simulink model "raibert_controller_1_3"  (R2018b)
settings: Solver=FixedStepDiscrete  StartTime=0.0  StopTime=inf  FixedStep=sample_time  RelTol=1e-3
InitFcn:
  | raibert_controller_params_1_3
  | warning off all
values from neighbouring files (symbols this model uses):
  sample_time = 1/sample_freq    (= 0.001)    [simulation_params.m]
undefined symbols (not defined in the file or in its folder): ctrl, Discrete, initial_dx_estimate, initial_dy_estimate, initial_dz_estimate, initial_z_estimate, Time
libraries: simulink x30, ctrlSharedLib x7
(part 1 of 4)
settings Model: Creator=wmartin  LastModifiedBy=akhadke
settings DataIOCC: SaveFormat=StructureWithTime  SaveOutput=off  SignalLogging=off  DSMLogging=off  SaveTime=off
settings OptimizationCC: BlockReduction=off  DefaultParameterBehavior=Inlined  UseFloatMulNetSlope=on  InlineInvariantSignals=on  OptimizeBlockIOStorage=off  BufferReuse=off  GlobalBufferReuse=off  ExpressionFolding=off  LocalBlockOutputs=off  LifeSpan=0.5  SimCompilerOptimization=on  OptimizeDataStoreBuffers=off  BusAssignmentInplaceUpdate=off
settings DebuggingCC: UnderspecifiedInitializationDetection=Classic  MergeDetectMultiDrivingBlocksExec=none  LibraryContextMissingDiagnostic=none
settings HardwareCC: ProdBitPerPointer=32  ProdBitPerSizeT=32  ProdBitPerPtrDiffT=32  ProdLargestAtomicFloat=None  ProdWordSize=32  ProdLongLongMode=on  ProdHWDeviceType=Generic->32-bit x86 compatible
settings ModelReferenceCC: ModelReferenceNumInstancesAllowed=Single  ModelReferenceMinAlgLoopOccurrences=on  PropagateSignalLabelsOutOfModel=off
settings SFSimCC: SimUseLocalCustomCode=off
settings RTWCC: SystemTargetFile=slrt.tlc  TLCOptions=-axPCModelStackSizeKB=1024  TemplateMakefile=slrt_default_tmf  Description=Simulink Real-Time  RTWUseLocalCustomCode=off  CodeExecutionProfiling=on  RTWCompilerOptimization=on
settings CodeAppCC: MaxIdLength=127  StateflowObjectComments=on
settings TargetCC: CodeReplacementLibrary=XPC_BLAS  ParMdlRefBuildCompliant=on  ConcurrentExecutionCompliant=on  GeneratePreprocessorConditionals=Use local settings  MatFileLogging=on  PreserveStateflowLocalDataDimensions=off  MATLABClassNameForMDSCustomization=xpcAperiodicCustomization

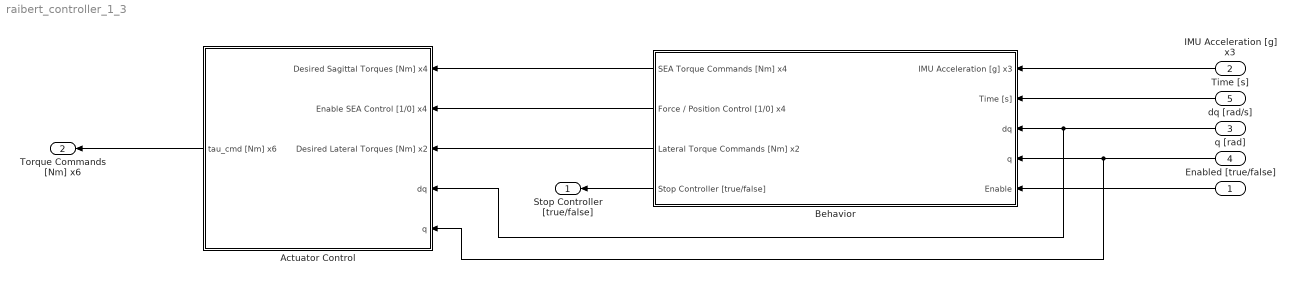
== system raibert_controller_1_3 ==
  Enabled [true/false] : Inport  OutDataTypeStr=boolean  PortDimensions=1  SampleTime=sample_time  Interpolate=off
  IMU Acceleration [g] x3 : Inport  Port=2  OutDataTypeStr=double  PortDimensions=3  SampleTime=sample_time  Interpolate=off
  dq [rad/s] : Inport  Port=3  OutDataTypeStr=double  PortDimensions=13  SampleTime=sample_time  Interpolate=off
  q [rad] : Inport  Port=4  OutDataTypeStr=double  PortDimensions=13  SampleTime=sample_time  Interpolate=off
  Time [s] : Inport  Port=5  OutDataTypeStr=double  PortDimensions=1  SampleTime=sample_time  Interpolate=off
  Actuator Control : Subsystem
  Behavior : Subsystem
  Stop Controller [true/false] : Outport  OutDataTypeStr=boolean  PortDimensions=1  SampleTime=[0.001,0]  OutputWhenDisabled=reset  InitialOutput=[0 0 0 0 0 0]
  Torque Commands [Nm] x6 : Outport  Port=2  OutDataTypeStr=double  PortDimensions=6  SampleTime=[0.001,0]  OutputWhenDisabled=reset  InitialOutput=[0 0 0 0 0 0]
  wires:
  IMU Acceleration [g] x3/1 -> Behavior/1(IMU Acceleration [g] x3)
  dq [rad/s]/1 -> Actuator Control/4(dq), Behavior/3(dq)
  q [rad]/1 -> Actuator Control/5(q), Behavior/4(q)
  Time [s]/1 -> Behavior/2(Time [s])
  Behavior/4(Stop Controller [true/false]) -> Stop Controller [true/false]/1
  Behavior/2(Force / Position Control [1/0] x4) -> Actuator Control/2(Enable SEA Control [1/0] x4)
  Actuator Control/1(tau_cmd [Nm] x6) -> Torque Commands [Nm] x6/1
  Behavior/1(SEA Torque Commands [Nm] x4) -> Actuator Control/1(Desired Sagittal Torques [Nm] x4)
  Behavior/3(Lateral Torque Commands [Nm] x2) -> Actuator Control/3(Desired Lateral Torques [Nm] x2)
  Enabled [true/false]/1 -> Behavior/5(Enable)

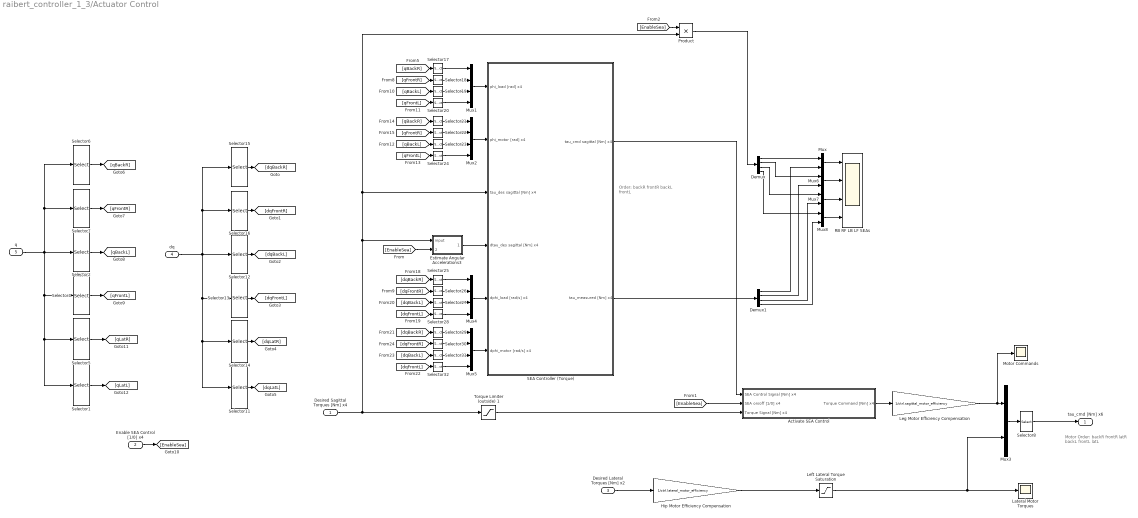
== system raibert_controller_1_3/Actuator Control ==
  note: Order:
      | backR
      | frontR
      | backL
      | frontL
  note: Motor Order:
      |
      | backR
      | frontR
      | latR
      | backL
      | frontL
      | latL
  Desired Sagittal Torques [Nm] x4 : Inport  OutDataTypeStr=double  PortDimensions=4  SampleTime=sample_time
  Enable SEA Control [1/0] x4 : Inport  Port=2  OutDataTypeStr=boolean  PortDimensions=4  SampleTime=sample_time
  Desired Lateral Torques [Nm] x2 : Inport  Port=3  OutDataTypeStr=double  PortDimensions=2  SampleTime=sample_time
  dq : Inport  Port=4  OutDataTypeStr=double  PortDimensions=13  SampleTime=sample_time
  q : Inport  Port=5  OutDataTypeStr=double  PortDimensions=13  SampleTime=sample_time
  Activate SEA Control : Subsystem
  Demux : Demux
  Demux1 : Demux
  Estimate Angular Accelerations3 : Subsystem
  Hip Motor Efficiency Compensation : Gain  Gain=1/ctrl.lateral_motor_efficiency
  Lateral Motor Torques : Scope
  Left Lateral Torque Saturation : Saturate  UpperLimit=ctrl.max_torque_lateral  LowerLimit=-ctrl.max_torque_lateral
      settings: AttributesFormatString=Top: %<UpperLimit>\nBottom: %<LowerLimit>
  Leg Motor Efficiency Compensation : Gain  Gain=1/ctrl.sagittal_motor_efficiency
  Motor Commands : Scope
  Mux{,3,6..8} (5 alike) : Mux  Inputs=2
  Mux{1..2,4..5} (4 alike) : Mux
  Product : Product
  RB RF LB LF SEAs : Scope  NumInputPorts=4
  SEA Controller (Torque) : Subsystem
  Selector1 : Selector  InputPortWidth=13  IndexOptions=Index vector (dialog)  Indices=[10]  OutputSizes=1
  Selector11 : Selector  InputPortWidth=13  IndexOptions=Index vector (dialog)  Indices=[10]  OutputSizes=1
  Selector12 : Selector  InputPortWidth=13  IndexOptions=Index vector (dialog)  Indices=[5 6]  OutputSizes=1
  Selector13 : Selector  InputPortWidth=13  IndexOptions=Index vector (dialog)  Indices=[7 8]  OutputSizes=1
  Selector14 : Selector  InputPortWidth=13  IndexOptions=Index vector (dialog)  Indices=[9]  OutputSizes=1
  Selector15 : Selector  InputPortWidth=13  IndexOptions=Index vector (dialog)  Indices=[1 2]  OutputSizes=1
  Selector16 : Selector  InputPortWidth=13  IndexOptions=Index vector (dialog)  Indices=[3 4]  OutputSizes=1
  Selector{17..20,25..28} (8 alike) : Selector  InputPortWidth=2  IndexOptions=Index vector (dialog)  Indices=[1]  OutputSizes=1
  Selector2 : Selector  InputPortWidth=13  IndexOptions=Index vector (dialog)  Indices=[5 6]  OutputSizes=1
  Selector{21..24,29..32} (8 alike) : Selector  InputPortWidth=2  IndexOptions=Index vector (dialog)  Indices=[2]  OutputSizes=1
  Selector4 : Selector  InputPortWidth=13  IndexOptions=Index vector (dialog)  Indices=[7 8]  OutputSizes=1
  Selector5 : Selector  InputPortWidth=13  IndexOptions=Index vector (dialog)  Indices=[9]  OutputSizes=1
  Selector6 : Selector  InputPortWidth=13  IndexOptions=Index vector (dialog)  Indices=[1 2]  OutputSizes=1
  Selector7 : Selector  InputPortWidth=13  IndexOptions=Index vector (dialog)  Indices=[3 4]  OutputSizes=1
  Selector8 : Selector  InputPortWidth=6  IndexOptions=Index vector (dialog)  Indices=[1 2 5 3 4 6]  OutputSizes=1
  Torque Limiter (outside) 1 : Saturate  UpperLimit=ctrl.max_sagittal_unloaded_torque  LowerLimit=-ctrl.max_sagittal_unloaded_torque
      settings: AttributesFormatString=Hi: %<UpperLimit>\nLo: %<LowerLimit>
  tau_cmd [Nm] x6 : Outport  OutDataTypeStr=double  PortDimensions=6  InitialOutput=[0 0 0 0 0 0]
  wires:
  Selector23/1 -> Mux2/3
  [qFrontL] -> Selector20/1
  Selector17/1 -> Mux1/1
  Selector19/1 -> Mux1/3
  Selector15/1 -> [dqBackR]
  [qFrontR] -> Selector18/1
  Selector13/1 -> [dqFrontL]
  [qBackR] -> Selector17/1
  Selector1/1 -> [qLatL]
  Mux1/1 -> SEA Controller (Torque)/1(phi_load [rad] x4)
  Selector12/1 -> [dqBackL]
  Torque Limiter (outside) 1/1 -> Activate SEA Control/3(Torque Signal [Nm] x4)
  [dqBackR] -> Selector25/1
  Selector29/1 -> Mux5/1
  Selector32/1 -> Mux5/4
  Mux5/1 -> SEA Controller (Torque)/6(dphi_motor [rad/s] x4)
  Mux4/1 -> SEA Controller (Torque)/5(dphi_load [rad/s] x4)
  Activate SEA Control/1(Torque Command [Nm] x4) -> Leg Motor Efficiency Compensation/1
  [dqFrontR] -> Selector26/1
  [qBackL] -> Selector23/1
  Selector25/1 -> Mux4/1
  Selector27/1 -> Mux4/3
  [dqFrontR] -> Selector30/1
  Selector24/1 -> Mux2/4
  Selector28/1 -> Mux4/4
  Estimate Angular Accelerations3/1(output) -> SEA Controller (Torque)/4(dtau_des sagittal [Nm] x4)
  [qFrontR] -> Selector22/1
  Selector22/1 -> Mux2/2
  [dqBackL] -> Selector27/1
  [EnableSea] -> Activate SEA Control/2("SEA on/off [1/0] x4 ")
  Selector30/1 -> Mux5/2
  [dqBackR] -> Selector29/1
  Selector31/1 -> Mux5/3
  Desired Lateral Torques [Nm] x2/1 -> Hip Motor Efficiency Compensation/1
  Selector2/1 -> [qBackL]
  Selector26/1 -> Mux4/2
  Mux3/1 -> Selector8/1
  [qFrontL] -> Selector24/1
  [dqFrontL] -> Selector28/1
  [dqBackL] -> Selector31/1
  [dqFrontL] -> Selector32/1
  Desired Sagittal Torques [Nm] x4/1 -> Estimate Angular Accelerations3/1(input), Product/2, SEA Controller (Torque)/3(tau_des sagittal [Nm] x4), Torque Limiter (outside) 1/1
  Selector4/1 -> [qFrontL]
  Selector18/1 -> Mux1/2
  Selector21/1 -> Mux2/1
  Selector5/1 -> [qLatR]
  [qBackR] -> Selector21/1
  SEA Controller (Torque)/2(tau_measured [Nm] x4) -> Demux1/1
  Selector20/1 -> Mux1/4
  Selector6/1 -> [qBackR]
  Selector8/1 -> tau_cmd [Nm] x6/1
  dq/1 -> Selector12/1, Selector16/1, Selector15/1, Selector13/1, Selector14/1, Selector11/1
  Selector11/1 -> [dqLatL]
  q/1 -> Selector1/1, Selector5/1, Selector4/1, Selector6/1, Selector7/1, Selector2/1
  Selector7/1 -> [qFrontR]
  [qBackL] -> Selector19/1
  Selector16/1 -> [dqFrontR]
  Selector14/1 -> [dqLatR]
  Mux2/1 -> SEA Controller (Torque)/2(phi_motor [rad] x4)
  Mux/1 -> RB RF LB LF SEAs/1
  Demux/1 -> Mux/1
  Demux1/1 -> Mux/2
  Mux6/1 -> RB RF LB LF SEAs/2
  Mux7/1 -> RB RF LB LF SEAs/3
  Mux8/1 -> RB RF LB LF SEAs/4
  Demux/2 -> Mux6/1
  Demux1/2 -> Mux6/2
  Demux/3 -> Mux7/1
  Demux1/3 -> Mux7/2
  Demux/4 -> Mux8/1
  Demux1/4 -> Mux8/2
  Enable SEA Control [1/0] x4/1 -> [EnableSea]
  [EnableSea] -> Product/1
  Product/1 -> Demux/1
  SEA Controller (Torque)/1(tau_cmd sagittal [Nm] x4) -> Activate SEA Control/1(SEA Control Signal [Nm] x4)
  Hip Motor Efficiency Compensation/1 -> Left Lateral Torque Saturation/1
  Leg Motor Efficiency Compensation/1 -> Motor Commands/1, Mux3/1
  Left Lateral Torque Saturation/1 -> Mux3/2, Lateral Motor Torques/1
  [EnableSea] -> Estimate Angular Accelerations3/2(enable [1/0])

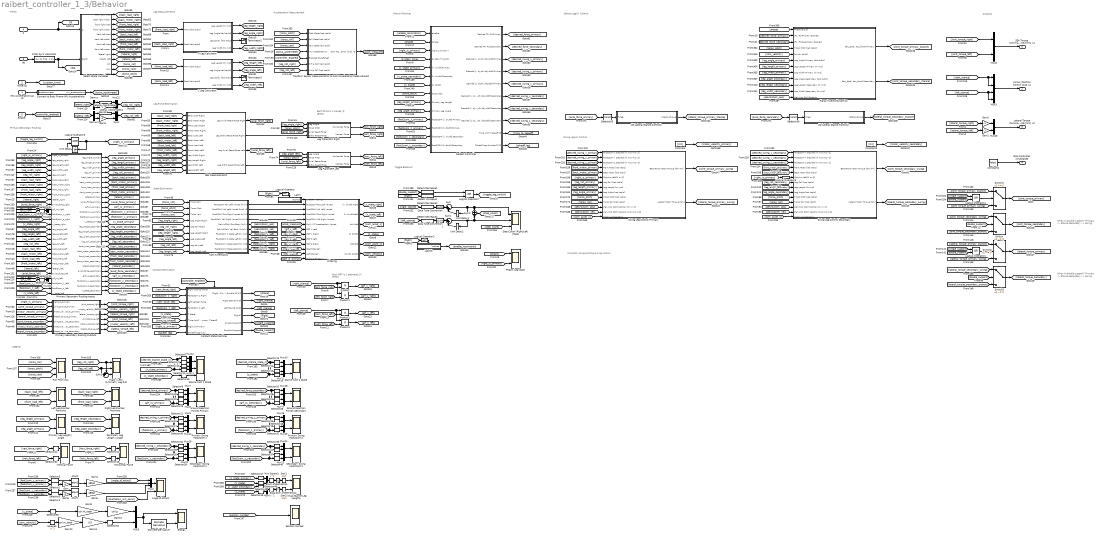
== system raibert_controller_1_3/Behavior ==
  note: Each GRF is 2 elements
      | [F, dF/dt]
  note: Primary/Secondary Routing
  note: Leg Measurements
  note: Outputs
  note: Inputs
  note: Contact Estimation
  note: Logging
  note: Acceleration Measurement
  note: Swing Leg(s) Control
  note: Leg Force Estimation
  note: Each force is 2 values
      | [F, dF/dt]
  note: State Estimation
  note: Toggle Behavior
  note: Motion Planning
  note: Stance Leg(s) Control
  note: Currently using existing swing control.
  note: When in double support?
      | Primary -> Stance
      | Secondary -> Swing
  note: When in double support?
      | Primary -> Stance
      | Secondary -> Swing
  IMU Acceleration [g] x3 : Inport  OutDataTypeStr=double  PortDimensions=3  SampleTime=[0.001,0]
  Time [s] : Inport  Port=2  OutDataTypeStr=double  PortDimensions=1  SampleTime=[0.001,0]
  dq : Inport  Port=3  OutDataTypeStr=double  PortDimensions=13  SampleTime=[0.001,0]
  q : Inport  Port=4  OutDataTypeStr=double  PortDimensions=13  SampleTime=[0.001,0]
  Enable : Inport  Port=5  OutDataTypeStr=boolean  PortDimensions=1  SampleTime=[0.001,0]
  2D Lateral Stance Control2 : MATLAB Function  TreatAsAtomicUnit=on
  2D Lateral Stance Control3 : MATLAB Function  TreatAsAtomicUnit=on
  Angle of Attack : Scope  NumInputPorts=2
  Atan1 : Trigonometry  Operator=atan2
  Atan2 : Trigonometry  Operator=atan2
  CoM Kinematics : Subsystem
  Constant : Constant  Value=[0 0]
  Constant2 : Constant  Value=false
  Constant5 : Constant  Value=[0 0]
  Contact State Machine : Subsystem
  Convert to Body Frame IMU Accelerations : MATLAB Function  TreatAsAtomicUnit=on
  Data Type Conversion : DataTypeConversion  OutDataTypeStr=double
  Data Type Conversion1 : DataTypeConversion  OutDataTypeStr=double
  Demux : Demux  Outputs=2
  Demux1 : Demux  Outputs=2
  Detect Decrease1 : simulink/Logic and Bit Operations/Detect Decrease  vinit=0  OutDataTypeStr=boolean
  Detect Decrease2 : simulink/Logic and Bit Operations/Detect Decrease  vinit=0  OutDataTypeStr=boolean
  Detect Decrease4 : simulink/Logic and Bit Operations/Detect Decrease  vinit=0  OutDataTypeStr=boolean
  Detect Increase2 : simulink/Logic and Bit Operations/Detect Increase  vinit=1  OutDataTypeStr=boolean
  Discrete Derivative : simulink/Discrete/Discrete Derivative  gainval=1.0  ICPrevScaledInput=0.0  OutMin=[]  OutMax=[]  OutDataType=fixdt(1, 16)  OutScaling=2^-10  DoSatur=off
  Energy : Scope  NumInputPorts=2
  Filter Gyro Velocities : Subsystem
  Filtering : Subsystem
  Gain{,1..3,6,12} (6 alike) : Gain  Gain=-1
  Gain10 : Gain  Gain=ctrl.m_total
  Gain11 : Gain  Gain=0.5
  Gain13 : Gain  Gain=ctrl.g
  Gain4 : Gain  Gain=180/pi
  Gain5 : Gain  Gain=180/pi
  Gain9 : Gain  Gain=ctrl.m_total
  Ground Reaction Forces Primary : Scope  NumInputPorts=2
  Ground Reaction Forces Secondary : Scope  NumInputPorts=2
  Horizontal Force : Scope  NumInputPorts=2
  L Leg Calculator : Subsystem
  Latch : Subsystem  TreatAsAtomicUnit=on
  Latch3 : Subsystem  TreatAsAtomicUnit=on
  Left Leg Fourbar Positions : Scope  NumInputPorts=2
  Leg Plane GRF Left : Subsystem
  Leg Plane GRF Right : Subsystem
  Logical Operator : Logic  Operator=NOT  AllPortsSameDT=off  OutDataTypeStr=boolean
  Logical Operator1 : Logic  Operator=OR  AllPortsSameDT=off  OutDataTypeStr=boolean
  Logical Operator2 : Logic  Operator=NOT  AllPortsSameDT=off  OutDataTypeStr=boolean
  Logical Operator3 : Logic  Operator=XOR  AllPortsSameDT=off  OutDataTypeStr=boolean
  Logical Operator4 : Logic  Operator=OR  AllPortsSameDT=off  OutDataTypeStr=boolean
  Logical Operator5 : Logic  Operator=NOT  AllPortsSameDT=off  OutDataTypeStr=boolean
  Logical Operator7 : Logic  Operator=OR  AllPortsSameDT=off  OutDataTypeStr=boolean
  Mux{,1,4..26} (25 alike) : Mux  Inputs=2
  Mux2 : Mux  Inputs=3
  Mux3 : Mux
  "Phase, Leg state" : Scope  NumInputPorts=2
  Planar Inverse Dynamics : Subsystem
  Primary Leg Length / Angle : Scope  NumInputPorts=2
  Primary Swing Foot2CoM X : Scope  NumInputPorts=2
  Primary Swing Foot2CoM Z : Scope  NumInputPorts=2
  Primary-Secondary Routing Inputs : MATLAB Function  TreatAsAtomicUnit=on
  Primary-Secondary Routing Outputs : MATLAB Function  TreatAsAtomicUnit=on
  Product{,1..3} (4 alike) : Product
  R Leg Calculator : Subsystem
  Raibert Controller : Subsystem
  Right / Left / Symmetry Leg Roll : Scope  NumInputPorts=3
  Right Leg Fourbar Positions : Scope  NumInputPorts=2
  Roll Pitch Yaw : Scope  NumInputPorts=3
  SEA Measurements : Subsystem
  Secondary Leg Length / Angle : Scope  NumInputPorts=2
  Secondary Swing Foot2CoM X : Scope  NumInputPorts=2
  Secondary Swing Foot2CoM Z : Scope  NumInputPorts=2
  Section Number : Scope
  Select State Variables : Subsystem
  Selector{10,12,15..16,21..23,28,30,32,38,40} (12 alike) : Selector  InputPortWidth=2  IndexOptions=Index vector (dialog)  Indices=[2]  OutputSizes=1
  Selector{11,18,34,36} (4 alike) : Selector  InputPortWidth=3  IndexOptions=Index vector (dialog)  Indices=[1]  OutputSizes=1
  Selector{2..9,13..14,20,24..27,29,31,33,39,41..52,55..56} (33 alike) : Selector  InputPortWidth=2  IndexOptions=Index vector (dialog)  Indices=[1]  OutputSizes=1
  Selector{17,19,35,37} (4 alike) : Selector  InputPortWidth=3  IndexOptions=Index vector (dialog)  Indices=[2]  OutputSizes=1
  Sqrt1 : Sqrt  SaturateOnIntegerOverflow=on
  Sqrt2 : Sqrt  SaturateOnIntegerOverflow=on
  Square1 : Math  Operator=square  SaturateOnIntegerOverflow=on
  Square2 : Math  Operator=square  SaturateOnIntegerOverflow=on
  Square3 : Math  Operator=square  SaturateOnIntegerOverflow=on
  Stance CoM X State : Scope  NumInputPorts=3
  Stance CoM Z State : Scope  NumInputPorts=2
  Step Count (Right/Left/Total) : Scope  NumInputPorts=3
  Sum : Sum  Inputs=|++
  Sum of Elements1 : Sum  Inputs=+
  Sum of Elements2 : Sum  Inputs=+
  Sum1 : Sum  Inputs=|++
  Sum2 : Sum  Inputs=+|+
  Sum3 : Sum  Inputs=-+|
  Swing Leg Control Primary : Subsystem
  Swing Leg Control Secondary : Subsystem
  Switch{,1..3} (4 alike) : Switch  Criteria=u2 ~= 0  Threshold=2
  Terminator2 : Terminator
  Terminator3 : Terminator
  Tranform Sensor Measurements to CoM Acceleration Measurement : Subsystem
  Unit Delay : UnitDelay  InitialCondition=ctrl.initial_leg_selection  SampleTime=sample_time
  Unit Delay1 : UnitDelay  SampleTime=-1
  Unit Delay2 : UnitDelay  SampleTime=-1
  Vertical Force : Scope  NumInputPorts=2
  Virtual Stance Leg Lengths : Scope  NumInputPorts=2
  lateral_coordinates : Fcn  Expr=pi/2-u
  lateral_coordinates1 : Fcn  Expr=pi/2-u
  SEA Torque Commands [Nm] x4 : Outport  OutDataTypeStr=double  PortDimensions=4  SampleTime=[0.001,0]  OutputWhenDisabled=reset  InitialOutput=[0 0 0 0]
  Force / Position Control [1/0] x4 : Outport  Port=2  OutDataTypeStr=boolean  PortDimensions=4  SampleTime=[0.001,0]  OutputWhenDisabled=reset  InitialOutput=[0 0 0 0]
  Lateral Torque Commands [Nm] x2 : Outport  Port=3  OutDataTypeStr=double  PortDimensions=2  SampleTime=[0.001,0]  OutputWhenDisabled=reset  InitialOutput=[0 0]
  Stop Controller [true/false] : Outport  Port=4  OutDataTypeStr=boolean  PortDimensions=1  SampleTime=[0.001,0]  OutputWhenDisabled=reset  InitialOutput=0
  wires:
  [leg_roll_right] -> Sum3/1, Right / Left / Symmetry Leg Roll/1
  [torso_pitch] -> Roll Pitch Yaw/2
  [leg_roll_left] -> Sum3/2, Right / Left / Symmetry Leg Roll/2
  Sum3/1 -> Right / Left / Symmetry Leg Roll/3
  [leg_length_primary] -> Primary Leg Length / Angle/1
  [leg_angle_primary] -> Primary Leg Length / Angle/2
  [leg_length_secondary] -> Secondary Leg Length / Angle/1
  [leg_angle_secondary] -> Secondary Leg Length / Angle/2
  [torso_roll] -> Roll Pitch Yaw/1
  [torso_yaw] -> Roll Pitch Yaw/3
  Time [s]/1 -> [system_time]
  Demux/2 -> Gain12/1
  lateral_coordinates/1 -> Mux22/1
  [back_load_left] -> Left Leg Fourbar Positions/1
  Gain12/1 -> Mux22/2
  [back_load_right] -> Right Leg Fourbar Positions/1
  Mux22/1 -> [leg_roll_right]
  Demux/1 -> lateral_coordinates/1
  [front_load_right] -> Right Leg Fourbar Positions/2
  [front_load_left] -> Left Leg Fourbar Positions/2
  [lateral_torque_right] -> Gain2/1
  L Leg Calculator/4(Leg Width [m m/s]) -> [leg_width_left]
  q/1 -> [q], Select State Variables/1(q)
  R Leg Calculator/4(Leg Width [m m/s]) -> [leg_width_right]
  L Leg Calculator/3(Leg Splay [rad rad/s]) -> Terminator3/1
  L Leg Calculator/2(Leg Angle [rad rad/s]) -> [leg_angle_left]
  L Leg Calculator/1("Leg Length [m m/s] ") -> [leg_length_left]
  R Leg Calculator/3(Leg Splay [rad rad/s]) -> Terminator2/1
  [lateral_torque_left] -> Gain1/1
  [back_load_right] -> R Leg Calculator/2(Back [rad rad/s])
  [front_load_right] -> R Leg Calculator/1(Front [rad rad/s])
  R Leg Calculator/2(Leg Angle [rad rad/s]) -> [leg_angle_right]
  R Leg Calculator/1("Leg Length [m m/s] ") -> [leg_length_right]
  [joint_torque_right] -> Mux8/1
  [joint_torque_left] -> Mux8/2
  Mux8/1 -> SEA Torque Commands [Nm] x4/1
  [left_stance] -> Mux3/3, Mux3/4
  [right_stance] -> Mux3/2, Mux3/1
  Mux3/1 -> Force / Position Control [1/0] x4/1
  Gain2/1 -> Mux25/1
  Mux25/1 -> Lateral Torque Commands [Nm] x2/1
  Gain1/1 -> Mux25/2
  [torso_pitch] -> Tranform Sensor Measurements to CoM Acceleration Measurement/1(Pitch State [rad rad/s])
  [torso_accelmeter] -> Tranform Sensor Measurements to CoM Acceleration Measurement/4(Imu Accelerations)
  [controller_enabled] -> Tranform Sensor Measurements to CoM Acceleration Measurement/5(Enabled [true/false])
  Tranform Sensor Measurements to CoM Acceleration Measurement/1(CoM Acceleration [m/s] x3) -> [accel_measure]
  [leg_roll_right] -> Tranform Sensor Measurements to CoM Acceleration Measurement/6(R Hip Roll [rad rad/s])
  [leg_roll_left] -> Tranform Sensor Measurements to CoM Acceleration Measurement/7(L Hip Roll [rad rad/s])
  [torso_roll] -> Tranform Sensor Measurements to CoM Acceleration Measurement/2(Roll State [rad rad/s])
  [torso_yaw] -> Tranform Sensor Measurements to CoM Acceleration Measurement/3(Yaw State [rad rad/s])
  Constant2/1 -> Stop Controller [true/false]/1
  dq/1 -> Filter Gyro Velocities/1(raw dq)
  Select State Variables/1(back right load) -> [back_load_right]
  Select State Variables/2(back right motor) -> [back_motor_right]
  Select State Variables/3(front right load) -> [front_load_right]
  Select State Variables/4(front right motor) -> [front_motor_right]
  Select State Variables/5(back left load) -> [back_load_left]
  Select State Variables/6(back left motor) -> [back_motor_left]
  Select State Variables/7(front left load) -> [front_load_left]
  Select State Variables/8(front left motor) -> [front_motor_left]
  Select State Variables/13(pitch) -> [torso_pitch]
  Select State Variables/12(yaw) -> [torso_yaw]
  Select State Variables/11(roll) -> [torso_roll]
  Select State Variables/10(lateral left) -> [lateral_left]
  Select State Variables/9(lateral right) -> [lateral_right]
  Logical Operator3/1 -> [right_is_primary], Unit Delay/1
  [toggle_leg_switch] -> Logical Operator3/1
  Unit Delay/1 -> Logical Operator3/2
  [front_load_left] -> L Leg Calculator/1(Front [rad rad/s])
  [back_load_left] -> L Leg Calculator/2(Back [rad rad/s])
  [lateral_right] -> Demux/1
  [lateral_left] -> Demux1/1
  Demux1/1 -> lateral_coordinates1/1
  Mux1/1 -> [leg_roll_left]
  Gain3/1 -> Mux1/2
  lateral_coordinates1/1 -> Mux1/1
  Demux1/2 -> Gain3/1
  Primary-Secondary Routing Inputs/1(leg_angle_primary) -> [leg_angle_primary]
  [leg_angle_right] -> Primary-Secondary Routing Inputs/2(leg_angle_right)
  [leg_length_right] -> Primary-Secondary Routing Inputs/3(leg_length_right)
  [leg_width_right] -> Primary-Secondary Routing Inputs/4(leg_width_right)
  [leg_roll_right] -> Primary-Secondary Routing Inputs/5(leg_roll_right)
  [back_load_right] -> Primary-Secondary Routing Inputs/6(back_load_right)
  [back_motor_right] -> Primary-Secondary Routing Inputs/7(back_motor_right)
  [front_load_right] -> Primary-Secondary Routing Inputs/8(front_load_right)
  [front_motor_right] -> Primary-Secondary Routing Inputs/9(front_motor_right)
  [lateral_right] -> Primary-Secondary Routing Inputs/10(lateral_right)
  [leg_angle_left] -> Primary-Secondary Routing Inputs/16(leg_angle_left)
  [leg_length_left] -> Primary-Secondary Routing Inputs/17(leg_length_left)
  [leg_width_left] -> Primary-Secondary Routing Inputs/18(leg_width_left)
  [leg_roll_left] -> Primary-Secondary Routing Inputs/19(leg_roll_left)
  [back_load_left] -> Primary-Secondary Routing Inputs/20(back_load_left)
  [back_motor_left] -> Primary-Secondary Routing Inputs/21(back_motor_left)
  [front_load_left] -> Primary-Secondary Routing Inputs/22(front_load_left)
  [front_motor_left] -> Primary-Secondary Routing Inputs/23(front_motor_left)
  [lateral_left] -> Primary-Secondary Routing Inputs/24(lateral_left)
  Primary-Secondary Routing Inputs/23(lateral_secondary) -> [lateral_secondary]
  Primary-Secondary Routing Inputs/22(front_motor_secondary) -> [front_motor_secondary]
  Primary-Secondary Routing Inputs/21(front_load_secondary) -> [front_load_secondary]
  Primary-Secondary Routing Inputs/20(back_motor_secondary) -> [back_motor_secondary]
  Primary-Secondary Routing Inputs/19(back_load_secondary) -> [back_load_secondary]
  Primary-Secondary Routing Inputs/18(leg_roll_secondary) -> [leg_roll_secondary]
  Primary-Secondary Routing Inputs/17(leg_width_secondary) -> [leg_width_secondary]
  Primary-Secondary Routing Inputs/16(leg_length_secondary) -> [leg_length_secondary]
  Primary-Secondary Routing Inputs/15(leg_angle_secondary) -> [leg_angle_secondary]
  Primary-Secondary Routing Inputs/9(lateral_primary) -> [lateral_primary]
  Primary-Secondary Routing Inputs/8(front_motor_primary) -> [front_motor_primary]
  Primary-Secondary Routing Inputs/7(front_load_primary) -> [front_load_primary]
  Primary-Secondary Routing Inputs/6(back_motor_primary) -> [back_motor_primary]
  Primary-Secondary Routing Inputs/5(back_load_primary) -> [back_load_primary]
  Primary-Secondary Routing Inputs/4(leg_roll_primary) -> [leg_roll_primary]
  Primary-Secondary Routing Inputs/3(leg_width_primary) -> [leg_width_primary]
  Primary-Secondary Routing Inputs/2(leg_length_primary) -> [leg_length_primary]
  Enable/1 -> [controller_enabled]
  Convert to Body Frame IMU Accelerations/1(imu_accelerations) -> [torso_accelmeter]
  IMU Acceleration [g] x3/1 -> Convert to Body Frame IMU Accelerations/1(accelerometer)
  [vert_force_right] -> Contact State Machine/1(Right Vertical Force)
  [vert_force_left] -> Contact State Machine/3(Left Vertical Force)
  [back_load_right] -> SEA Measurements/1(Back Load Right)
  [back_motor_right] -> SEA Measurements/2(Back Motor Right)
  [front_load_right] -> SEA Measurements/3(Front Load Right)
  [front_motor_right] -> SEA Measurements/4(Front Motor Right)
  [back_load_left] -> SEA Measurements/5(Back Load Left)
  [back_motor_left] -> SEA Measurements/6(Back Motor Left)
  [front_load_left] -> SEA Measurements/7(Front Load Left)
  [front_motor_left] -> SEA Measurements/8(Front Motor Left)
  [leg_width_right] -> SEA Measurements/9(Leg Width Right)
  [leg_length_left] -> SEA Measurements/12(Leg Length Left)
  [leg_length_right] -> SEA Measurements/10(Leg Length Right)
  [leg_width_left] -> SEA Measurements/11(Leg Width Left)
  SEA Measurements/2(Leg Ortho React Force Right) -> Leg Plane GRF Right/4(Ortho React Force)
  [torso_pitch] -> Leg Plane GRF Right/2(Torso Pitch)
  [leg_angle_right] -> Leg Plane GRF Right/1(Leg Angle)
  [leg_angle_left] -> Leg Plane GRF Left/1(Leg Angle)
  [torso_pitch] -> Leg Plane GRF Left/2(Torso Pitch)
  Leg Plane GRF Right/2(Vertical Force) -> [vert_force_right]
  [vert_force_right] -> Selector44/1
  [vert_force_left] -> Selector52/1
  [horz_force_right] -> Selector42/1
  [horz_force_left] -> Selector43/1
  [torso_pitch] -> CoM Kinematics/2(Torso Pitch)
  [torso_roll] -> CoM Kinematics/1(Torso Roll)
  [torso_yaw] -> CoM Kinematics/3(Torso Yaw)
  [leg_length_left] -> CoM Kinematics/9(Leg Length Left)
  [leg_length_right] -> CoM Kinematics/6(Leg Length Right)
  [leg_angle_right] -> CoM Kinematics/4(Leg Angle Right)
  [leg_angle_left] -> CoM Kinematics/7(Leg Angle Left)
  [leg_roll_left] -> CoM Kinematics/8(Leg Roll Left)
  [leg_roll_right] -> CoM Kinematics/5(Leg Roll Right)
  [horz_force_right] -> Product/2
  [vert_force_right] -> Product1/2
  [right_stance] -> Product1/1, Product/1
  [vert_force_left] -> Product3/2
  [horz_force_left] -> Product2/2
  [left_stance] -> Product3/1, Product2/1
  Product/1 -> [grf_x_right]
  Product1/1 -> [grf_z_right]
  Product2/1 -> [grf_x_left]
  Product3/1 -> [grf_z_left]
  CoM Kinematics/1(Foot2CoM Pos Left Yawed [m] x3) -> Filtering/2(Foot2CoM Pos Left Yawed)
  CoM Kinematics/2(Foot2CoM Vel Left Yawed [m/s] x3) -> Filtering/3(Foot2CoM Vel Left Yawed)
  CoM Kinematics/3(Foot2CoM Pos Right Yawed [m] x3) -> Filtering/4(Foot2CoM Pos Right Yawed)
  CoM Kinematics/4(Foot2CoM Vel Right Yawed [m/s] x3) -> Filtering/5(Foot2CoM Vel Right Yawed)
  [accel_measure] -> Filtering/6(CoM XYZ Acceleration Yawed)
  [grf_x_left] -> Filtering/7(GRF X Left)
  [grf_x_right] -> Filtering/8(GRF X Right)
  [grf_z_left] -> Filtering/9(GRF Z Left)
  [grf_z_right] -> Filtering/10(GRF Z Right)
  [right_stance] -> Filtering/11(Right Stance?)
  [left_stance] -> Filtering/12(Left Stance?)
  [right_is_primary] -> Filtering/13(Right Is Primary?)
  Filtering/1("[x, dx/dt] Right") -> [x_state_right]
  Filtering/2("[x, dx/dt] Left") -> [x_state_left]
  Filtering/3(ddx/ddt) -> [com_accel_x]
  Filtering/4("[z, dz/dt]") -> [z_state]
  Filtering/5(ddz/ddt) -> [com_accel_z]
  [flight] -> Logical Operator/1
  Logical Operator/1 -> Latch/Enable
  Contact State Machine/1(Flight / Single / Double [0/1/2]) -> [phase]
  Latch/1(latched) -> Filtering/1(Enable Filtering)
  CoM Kinematics/5(Pelvis2CoM Pos Body [m] x3) -> [pelvis2com_pos]
  CoM Kinematics/6(Pelvis2CoM Vel Body [m/s] x3) -> [pelvis2com_vel]
  Primary-Secondary Routing Outputs/1(joint_torque_right) -> [joint_torque_right]
  Primary-Secondary Routing Outputs/2(motor_velocity_right) -> [motor_velcoity_right]
  Primary-Secondary Routing Outputs/6(lateral_torque_left) -> [lateral_torque_left]
  Primary-Secondary Routing Outputs/5(motor_velocity_left) -> [motor_velocity_left]
  Primary-Secondary Routing Outputs/4(joint_torque_left) -> [joint_torque_left]
  Primary-Secondary Routing Outputs/3(lateral_torque_right) -> [lateral_torque_right]
  [joint_torque_secondary] -> Primary-Secondary Routing Outputs/5(joint_torque_secondary)
  [motor_velocity_secondary] -> Primary-Secondary Routing Outputs/6(motor_velocity_secondary)
  [lateral_torque_secondary] -> Primary-Secondary Routing Outputs/7(lateral_torque_secondary)
  [lateral_torque_primary] -> Primary-Secondary Routing Outputs/4(lateral_torque_primary)
  [motor_velocity_primary] -> Primary-Secondary Routing Outputs/3(motor_velocity_primary)
  [joint_torque_primary] -> Primary-Secondary Routing Outputs/2(joint_torque_primary)
  [right_is_primary] -> Primary-Secondary Routing Inputs/1(right_is_primary)
  [right_is_primary] -> Primary-Secondary Routing Outputs/1(right_is_primary)
  Filtering/6("[dx/dt, dz/dt]") -> [com_velocity]
  [desired_swing_x_secondary] -> Swing Leg Control Secondary/1(Foot2CoM X Desired [m m/s m/s^2])
  [desired_swing_z_secondary] -> Swing Leg Control Secondary/3(Foot2CoM Z Desired [m m/s m/s^2])
  [pelvis2com_vel] -> Swing Leg Control Secondary/13(Pelvis to COM Velocity [m/s m/s m/s])
  [pelvis2com_pos] -> Swing Leg Control Secondary/12(Pelvis to COM Position [m m m])
  [torso_pitch] -> Swing Leg Control Secondary/10(Torso Pitch [rad rad/s])
  [torso_roll] -> Swing Leg Control Secondary/11(Torso Roll [rad rad/s])
  [right_is_primary] -> Logical Operator5/1
  [back_motor_secondary] -> Swing Leg Control Secondary/5(Back Motor [rad rad/s])
  [front_motor_secondary] -> Swing Leg Control Secondary/4(Front Motor [rad rad/s])
  [leg_roll_secondary] -> Swing Leg Control Secondary/7(Leg Roll [rad rad/s])
  [leg_length_secondary] -> Swing Leg Control Secondary/8(Leg Length [m m/s])
  [leg_angle_secondary] -> Swing Leg Control Secondary/9(Leg Angle [rad rad/s])
  Switch/1 -> [joint_torque_secondary]
  [double_support] -> Switch/2
  [desired_swing_y_secondary] -> Swing Leg Control Secondary/2(Foot2CoM Y Desired [m m/s m/s^2])
  SEA Measurements/1(Leg Axial React Force Right) -> [axial_force_right]
  SEA Measurements/3(Leg Axial React Force Left) -> [axial_force_left]
  [axial_force_right] -> Leg Plane GRF Right/3(Axial React Force)
  [axial_force_left] -> Leg Plane GRF Left/3(Axial React Force)
  [axial_force_right] -> Primary-Secondary Routing Inputs/11(axial_force_right)
  [axial_force_left] -> Primary-Secondary Routing Inputs/25(axial_force_left)
  Primary-Secondary Routing Inputs/24(axial_force_secondary) -> [axial_force_secondary]
  Primary-Secondary Routing Inputs/10(axial_force_primary) -> [axial_force_primary]
  [single_support] -> Logical Operator1/1
  [double_support] -> Logical Operator1/2
  Logical Operator1/1 -> Switch2/2
  Switch2/1 -> [lateral_torque_primary]
  [joint_torque_secondary_swing] -> Switch/1
  Swing Leg Control Secondary/1(Back/Front Motor Torque [Nm Nm]) -> [joint_torque_secondary_swing]
  [joint_torque_secondary_stance] -> Switch/3
  [lateral_torque_primary_stance] -> Switch2/1
  [lateral_torque_primary_swing] -> Switch2/3
  Switch3/1 -> [lateral_torque_secondary]
  [double_support] -> Switch3/2
  Swing Leg Control Secondary/2(Lateral Motor Torque [Nm]) -> [lateral_torque_secondary_swing]
  [lateral_torque_secondary_swing] -> Switch3/1
  [lateral_torque_secondary_stance] -> Switch3/3
  [joint_torque_primary_swing] -> Switch1/3
  [joint_torque_primary_stance] -> Switch1/1
  Logical Operator4/1 -> Switch1/2
  Switch1/1 -> [joint_torque_primary]
  [double_support] -> Logical Operator4/2
  [single_support] -> Logical Operator4/1
  [com_accel_z] -> Swing Leg Control Secondary/14(CoM Z Acceleration)
  [com_accel_z] -> Swing Leg Control Primary/14(CoM Z Acceleration)
  [desired_swing_y_primary] -> Swing Leg Control Primary/2(Foot2CoM Y Desired [m m/s m/s^2])
  [leg_angle_primary] -> Swing Leg Control Primary/9(Leg Angle [rad rad/s])
  [leg_length_primary] -> Swing Leg Control Primary/8(Leg Length [m m/s])
  [leg_roll_primary] -> Swing Leg Control Primary/7(Leg Roll [rad rad/s])
  [front_motor_primary] -> Swing Leg Control Primary/4(Front Motor [rad rad/s])
  [back_motor_primary] -> Swing Leg Control Primary/5(Back Motor [rad rad/s])
  [right_is_primary] -> Swing Leg Control Primary/6(Right or Left [1 or 0])
  [torso_roll] -> Swing Leg Control Primary/11(Torso Roll [rad rad/s])
  [torso_pitch] -> Swing Leg Control Primary/10(Torso Pitch [rad rad/s])
  [pelvis2com_pos] -> Swing Leg Control Primary/12(Pelvis to COM Position [m m m])
  [pelvis2com_vel] -> Swing Leg Control Primary/13(Pelvis to COM Velocity [m/s m/s m/s])
  [desired_swing_z_primary] -> Swing Leg Control Primary/3(Foot2CoM Z Desired [m m/s m/s^2])
  [desired_swing_x_primary] -> Swing Leg Control Primary/1(Foot2CoM X Desired [m m/s m/s^2])
  Swing Leg Control Primary/1(Back/Front Motor Torque [Nm Nm]) -> [joint_torque_primary_swing]
  Swing Leg Control Primary/2(Lateral Motor Torque [Nm]) -> [lateral_torque_primary_swing]
  Logical Operator5/1 -> Swing Leg Control Secondary/6(Right or Left [1 or 0])
  [x_state_right] -> Primary-Secondary Routing Inputs/15(x_state_right)
  [x_state_left] -> Primary-Secondary Routing Inputs/29(x_state_left)
  Primary-Secondary Routing Inputs/14(x_state_primary) -> [x_state_primary]
  Primary-Secondary Routing Inputs/28(x_state_secondary) -> [x_state_secondary]
  Leg Plane GRF Right/1(Horizontal Force) -> [horz_force_right]
  Leg Plane GRF Left/1(Horizontal Force) -> [horz_force_left]
  Leg Plane GRF Left/2(Vertical Force) -> [vert_force_left]
  SEA Measurements/4(Leg Ortho React Force Left) -> Leg Plane GRF Left/4(Ortho React Force)
  [double_support] -> Detect Decrease1/1
  [flight] -> Detect Increase2/1
  [desired_stance_state_z] -> Selector15/1, Selector13/1
  Selector12/1 -> Mux13/2
  Mux11/1 -> Stance CoM Z State/2
  Selector13/1 -> Mux10/1
  Mux10/1 -> Stance CoM Z State/1
  Selector6/1 -> Mux12/1
  Selector14/1 -> Mux10/2
  [z_state] -> Selector14/1, Selector16/1
  [x_state_primary] -> Selector7/1, Selector12/1
  Selector16/1 -> Mux11/2
  Mux13/1 -> Stance CoM X State/2
  Selector15/1 -> Mux11/1
  Selector7/1 -> Mux12/2
  Selector10/1 -> Mux13/1
  Mux12/1 -> Stance CoM X State/1
  [desired_stance_state_x] -> Selector6/1, Selector10/1
  Mux9/1 -> Primary Swing Foot2CoM X/1
  Mux14/1 -> Primary Swing Foot2CoM X/2
  [desired_swing_x_primary] -> Selector17/1, Selector11/1
  Selector11/1 -> Mux9/1
  Selector17/1 -> Mux14/1
  Selector19/1 -> Mux15/1
  Selector18/1 -> Mux16/1
  [desired_swing_z_primary] -> Selector18/1, Selector19/1
  Mux15/1 -> Primary Swing Foot2CoM Z/2
  Mux16/1 -> Primary Swing Foot2CoM Z/1
  CoM Kinematics/7(Foot2CoM X State Left [m m/s]) -> [foot2com_x_left]
  CoM Kinematics/8(Foot2CoM Z State Left [m m/s]) -> [foot2com_z_left]
  CoM Kinematics/9(Foot2CoM X State Right [m m/s]) -> [foot2com_x_right]
  CoM Kinematics/10(Foot2CoM Z State Right [m m/s]) -> [foot2com_z_right]
  Mux6/1 -> Ground Reaction Forces Primary/2
  Mux7/1 -> Ground Reaction Forces Primary/1
  [desired_force_primary] -> Selector22/1, Selector8/1
  Selector8/1 -> Mux7/1
  Selector22/1 -> Mux6/1
  Selector21/1 -> Mux17/1
  [desired_force_secondary] -> Selector21/1, Selector20/1
  Selector20/1 -> Mux18/1
  Mux18/1 -> Ground Reaction Forces Secondary/1
  Mux17/1 -> Ground Reaction Forces Secondary/2
  [grf_z_right] -> Selector24/1
  [grf_x_right] -> Selector9/1
  [foot2com_x_right] -> Primary-Secondary Routing Inputs/13(foot2com_x_right)
  [foot2com_z_right] -> Primary-Secondary Routing Inputs/14(foot2com_z_right)
  [foot2com_x_left] -> Primary-Secondary Routing Inputs/27(foot2com_x_left)
  [foot2com_z_left] -> Primary-Secondary Routing Inputs/28(foot2com_z_left)
  Selector9/1 -> Mux19/1
  Selector24/1 -> Mux19/2
  Mux19/1 -> Primary-Secondary Routing Inputs/12(grf_xz_right)
  Selector26/1 -> Mux20/2
  Selector27/1 -> Mux20/1
  [grf_x_left] -> Selector27/1
  Mux20/1 -> Primary-Secondary Routing Inputs/26(grf_xz_left)
  [grf_z_left] -> Selector26/1
  Primary-Secondary Routing Inputs/12(foot2com_x_primary) -> [foot2com_x_primary]
  Primary-Secondary Routing Inputs/13(foot2com_z_primary) -> [foot2com_z_primary]
  Primary-Secondary Routing Inputs/11(grf_xz_primary) -> [grf_xz_primary]
  Primary-Secondary Routing Inputs/25(grf_xz_secondary) -> [grf_xz_secondary]
  Primary-Secondary Routing Inputs/26(foot2com_x_secondary) -> [foot2com_x_secondary]
  Primary-Secondary Routing Inputs/27(foot2com_z_secondary) -> [foot2com_z_secondary]
  Selector25/1 -> Mux7/2
  Selector23/1 -> Mux6/2
  [grf_xz_primary] -> Selector25/1, Selector23/1
  Selector29/1 -> Mux18/2
  Selector28/1 -> Mux17/2
  [grf_xz_secondary] -> Selector28/1, Selector29/1
  Selector31/1 -> Mux9/2
  Selector30/1 -> Mux14/2
  [foot2com_x_primary] -> Selector30/1, Selector31/1
  Selector33/1 -> Mux16/2
  Selector32/1 -> Mux15/2
  [foot2com_z_primary] -> Selector33/1, Selector32/1
  [foot2com_z_secondary] -> Selector40/1, Selector41/1
  Selector40/1 -> Mux23/2
  Selector41/1 -> Mux24/2
  [foot2com_x_secondary] -> Selector39/1, Selector38/1
  Selector38/1 -> Mux21/2
  Selector39/1 -> Mux26/2
  Mux24/1 -> Secondary Swing Foot2CoM Z/1
  Mux23/1 -> Secondary Swing Foot2CoM Z/2
  [desired_swing_z_secondary] -> Selector37/1, Selector36/1
  Selector36/1 -> Mux24/1
  Selector37/1 -> Mux23/1
  Selector35/1 -> Mux21/1
  Selector34/1 -> Mux26/1
  [desired_swing_x_secondary] -> Selector34/1, Selector35/1
  Mux21/1 -> Secondary Swing Foot2CoM X/2
  Mux26/1 -> Secondary Swing Foot2CoM X/1
  [angle_of_attack] -> Mux2/1
  [touchdown_will_occur] -> Angle of Attack/2
  Mux2/1 -> Angle of Attack/1
  Atan2/1 -> Gain4/1
  [foot2com_z_primary] -> Selector3/1
  [foot2com_x_primary] -> Selector2/1
  Selector2/1 -> Gain/1
  Gain4/1 -> Mux2/2
  Selector3/1 -> Atan2/1
  Gain/1 -> Atan2/2
  Gain5/1 -> Mux2/3
  Gain6/1 -> Atan1/2
  Selector5/1 -> Atan1/1
  Selector4/1 -> Gain6/1
  Atan1/1 -> Gain5/1
  [foot2com_x_secondary] -> Selector4/1
  [foot2com_z_secondary] -> Selector5/1
  Logical Operator7/1 -> [toggle_leg_switch]
  [z_state] -> Contact State Machine/5(Z State)
  [foot2com_z_left] -> Contact State Machine/4(Foot2Com Z Left)
  [foot2com_z_right] -> Contact State Machine/2(Foot2Com Z Right)
  Detect Decrease1/1 -> Logical Operator7/1
  Detect Increase2/1 -> Logical Operator7/2
  [x_state_secondary] -> Selector45/1
  Selector45/1 -> Stance CoM X State/3
  Sum of Elements1/1 -> Sqrt1/1
  Square1/1 -> Sum of Elements1/1
  [x_state_primary] -> Selector47/1
  [z_state] -> Selector48/1
  Selector47/1 -> Mux/1
  Selector48/1 -> Mux/2
  Mux/1 -> Square1/1
  Sqrt1/1 -> Virtual Stance Leg Lengths/1
  Sqrt2/1 -> Virtual Stance Leg Lengths/2
  Mux4/1 -> Square2/1
  Selector49/1 -> Mux4/2
  [z_state] -> Selector49/1
  Square2/1 -> Sum of Elements2/1
  Sum of Elements2/1 -> Sqrt2/1
  [x_state_secondary] -> Selector46/1
  Selector46/1 -> Mux4/1
  [time_to_takeoff] -> Contact State Machine/6(Time Untill Primary Takeoff)
  [right_is_primary] -> Contact State Machine/7(Right is Primary?)
  [z_state] -> Selector50/1
  [com_velocity] -> Square3/1
  Selector50/1 -> Gain9/1
  Square3/1 -> Gain10/1
  Gain10/1 -> Gain11/1
  Gain11/1 -> Selector51/1
  Gain9/1 -> Gain13/1
  Gain13/1 -> Mux5/1
  Mux5/1 -> Energy/1, Discrete Derivative/1
  Discrete Derivative/1 -> Energy/2
  Selector42/1 -> Horizontal Force/1
  Selector43/1 -> Horizontal Force/2
  Selector44/1 -> Vertical Force/1
  Selector52/1 -> Vertical Force/2
  Selector51/1 -> Mux5/2
  [takeoff_leg] -> Contact State Machine/8(Takeoff Leg [1/2])
  [section_number] -> Section Number/1
  [right_stance] -> Detect Decrease2/1
  [left_stance] -> Detect Decrease4/1
  Detect Decrease2/1 -> Data Type Conversion/1
  Unit Delay1/1 -> Sum/2
  Sum/1 -> Unit Delay1/1, Step Count (Right/Left/Total)/1, Sum2/1
  Sum1/1 -> Sum2/2, Step Count (Right/Left/Total)/2, Unit Delay2/1
  Unit Delay2/1 -> Sum1/2
  Detect Decrease4/1 -> Data Type Conversion1/1
  Data Type Conversion/1 -> Sum/1
  Data Type Conversion1/1 -> Sum1/1
  Sum2/1 -> [step_count]
  [step_count] -> Step Count (Right/Left/Total)/3
  Planar Inverse Dynamics/2("[tau_back, tau_front] Secondary") -> [joint_torque_secondary_stance]
  Selector56/1 -> 2D Lateral Stance Control2/1(F_leg)
  [phase] -> Planar Inverse Dynamics/1(Phase [0/1/2])
  Selector55/1 -> 2D Lateral Stance Control3/1(F_leg)
  [leg_length_primary] -> Planar Inverse Dynamics/7(Leg Length Primary [m m/s])
  [com_velocity] -> Planar Inverse Dynamics/5("[dx/dt, dz/dt]")
  [axial_force_primary] -> Selector55/1
  [leg_length_secondary] -> Planar Inverse Dynamics/10(Leg Length Secondary [m m/s])
  [leg_angle_primary] -> Planar Inverse Dynamics/6(Leg Angle Primary [rad rad/s])
  [torso_pitch] -> Planar Inverse Dynamics/4(Torso Pitch [rad rad/s])
  [leg_angle_secondary] -> Planar Inverse Dynamics/9(Leg Angle Secondary [rad rad/s])
  [leg_width_primary] -> Planar Inverse Dynamics/8(Leg Width Primary [m m/s])
  2D Lateral Stance Control3/1(lateral_torque) -> [lateral_torque_primary_stance]
  [pelvis2com_pos] -> Planar Inverse Dynamics/12(Pelvis to CoM Position)
  Planar Inverse Dynamics/1("[tau_back, tau_front] Primary") -> [joint_torque_primary_stance]
  [leg_width_secondary] -> Planar Inverse Dynamics/11(Leg Width Secondary [m m/s])
  [axial_force_secondary] -> Selector56/1
  2D Lateral Stance Control2/1(lateral_torque) -> [lateral_torque_secondary_stance]
  [controller_enabled] -> Contact State Machine/Enable
  Constant/1 -> [motor_velocity_primary]
  Constant5/1 -> [motor_velocity_secondary]
  Contact State Machine/2(Right Stance [1/0]) -> [right_stance]
  Contact State Machine/3(Left Stance [1/0]) -> [left_stance]
  Contact State Machine/4(Flight?) -> [flight]
  Contact State Machine/5(Single Support?) -> [single_support]
  Contact State Machine/6(Double Support?) -> [double_support]
  Filter Gyro Velocities/1(filtered dq) -> [dq], Select State Variables/2(dq/dt)
  Logical Operator2/1 -> Latch3/Enable
  [flight] -> Logical Operator2/1
  Latch3/1(latched) -> [enable_locomotion]
  [torso_pitch] -> Raibert Controller/8(torso pitch)
  Raibert Controller/3("Desired [x, dx/dt, ddx/ddt] Primary") -> [desired_swing_x_primary]
  Raibert Controller/4("Desired [y, dy/dt, ddy/ddt] Primary") -> [desired_swing_y_primary]
  Raibert Controller/7("Desired [y, dy/dt, ddy/ddt] Secondary") -> [desired_swing_y_secondary]
  [foot2com_z_primary] -> Raibert Controller/12("foot2COM [z, dz/dt] Primary")
  Raibert Controller/6("Desired [x, dx/dt, ddx/ddt] Secondary") -> [desired_swing_x_secondary]
  Raibert Controller/8("Desired [z, dz/dt, ddz/ddt] Secondary") -> [desired_swing_z_secondary]
  Raibert Controller/1(Desired [Fx Fz] Primary) -> [desired_force_primary]
  Raibert Controller/5("Desired [z, dz/dt, ddz/ddt] Primary") -> [desired_swing_z_primary]
  Raibert Controller/2(Desired [Fx Fz] Secondary) -> [desired_force_secondary]
  [foot2com_x_primary] -> Raibert Controller/11("foot2COM [x, dx/dt] Primary")
  [foot2com_x_secondary] -> Raibert Controller/13("foot2COM [x, dx/dt] Secondary")
  [foot2com_z_secondary] -> Raibert Controller/14("foot2COM [z, dz/dt] Secondary")
  [x_state_primary] -> Raibert Controller/5("[x, dx/dt] Primary")
  [x_state_secondary] -> Raibert Controller/6("[x, dx/dt] Secondary")
  [z_state] -> Raibert Controller/7("[z, dz/dt]")
  Raibert Controller/9(TIme Until Takeoff [s]) -> [time_to_takeoff]
  Raibert Controller/10(Takeoff Leg Number [1/2]) -> [takeoff_leg]
  [right_is_primary] -> Raibert Controller/3(right is primary?)
  [system_time] -> Raibert Controller/4(System Time [s])
  [enable_locomotion] -> Raibert Controller/1(enable)
  [phase] -> Raibert Controller/2(phase)
  [desired_force_primary] -> Planar Inverse Dynamics/2("[Fx, Fz] Primary Desired")
  [desired_force_secondary] -> Planar Inverse Dynamics/3("[Fx, Fz] Secondary Desired")
  [phase] -> "Phase, Leg state"/1
  [right_is_primary] -> "Phase, Leg state"/2
  [leg_length_primary] -> Raibert Controller/9(Primary Leg Length)
  [leg_angle_primary] -> Raibert Controller/10(Primary Leg Angle)

== system raibert_controller_1_3/Actuator Control/Activate SEA Control ==
  SEA Control Signal [Nm] x4 : Inport
  "SEA on/off [1/0] x4 " : Inport  Port=2
  Torque Signal [Nm] x4 : Inport  Port=3
  Demux : Demux
  Demux2 : Demux
  Demux3 : Demux
  Mux6 : Mux
  Switch{,1..3} (4 alike) : Switch  Criteria=u2 ~= 0
  Torque Command [Nm] x4 : Outport
  wires:
  Torque Signal [Nm] x4/1 -> Demux2/1
  "SEA on/off [1/0] x4 "/1 -> Demux3/1
  SEA Control Signal [Nm] x4/1 -> Demux/1
  Demux2/3 -> Switch2/3
  Demux/2 -> Switch1/1
  Demux3/4 -> Switch3/2
  Demux2/4 -> Switch3/3
  Demux/4 -> Switch3/1
  Switch2/1 -> Mux6/3
  Demux/3 -> Switch2/1
  Demux3/2 -> Switch1/2
  Demux3/3 -> Switch2/2
  Mux6/1 -> Torque Command [Nm] x4/1
  Demux3/1 -> Switch/2
  Switch3/1 -> Mux6/4
  Switch1/1 -> Mux6/2
  Switch/1 -> Mux6/1
  Demux/1 -> Switch/1
  Demux2/1 -> Switch/3
  Demux2/2 -> Switch1/3

== system raibert_controller_1_3/Actuator Control/Estimate Angular Accelerations3 ==
  input : Inport
  enable [1/0] : Inport  Port=2
  Demux : Demux
  Demux1 : Demux
  Detect Change : simulink/Logic and Bit Operations/Detect Change  vinit=0  OutDataTypeStr=boolean
  Difference : simulink/Discrete/Difference  ICPrevInput=0.0  OutMin=[]  OutMax=[]  OutDataType=fixdt(1, 16)  OutScaling=2^-10  DoSatur=off
  Gain : Gain  Gain=1/sample_time
  IMU Two Pole Filter{,1..3} (4 alike) : DiscreteTransferFcn  Numerator=[ctrl.A_lpf_dtau 0 0]  Denominator=[1 ctrl.B1_lpf_dtau ctrl.B2_lpf_dtau]  ExternalReset=Rising  SampleTime=sample_time
      settings: InputPortMap=u0,r7
  Logical Operator : Logic  Operator=NOT  AllPortsSameDT=off  OutDataTypeStr=boolean
  Mux : Mux
  Product : Product
  output : Outport
  wires:
  input/1 -> Difference/1
  Difference/1 -> Product/1
  Product/1 -> Gain/1
  Detect Change/1 -> Logical Operator/1
  Logical Operator/1 -> Product/2
  Gain/1 -> Demux/1
  IMU Two Pole Filter/1 -> Mux/1
  IMU Two Pole Filter1/1 -> Mux/2
  IMU Two Pole Filter2/1 -> Mux/3
  IMU Two Pole Filter3/1 -> Mux/4
  Demux/1 -> IMU Two Pole Filter/1
  Demux/2 -> IMU Two Pole Filter1/1
  Demux/3 -> IMU Two Pole Filter2/1
  Demux/4 -> IMU Two Pole Filter3/1
  Demux1/1 -> IMU Two Pole Filter/2
  Demux1/2 -> IMU Two Pole Filter1/2
  Demux1/3 -> IMU Two Pole Filter2/2
  Demux1/4 -> IMU Two Pole Filter3/2
  enable [1/0]/1 -> Demux1/1, Detect Change/1
  Mux/1 -> output/1

== system raibert_controller_1_3/Actuator Control/SEA Controller (Torque) ==
  phi_load [rad] x4 : Inport
  phi_motor [rad] x4 : Inport  Port=2
  tau_des sagittal [Nm] x4 : Inport  Port=3
  dtau_des sagittal [Nm] x4 : Inport  Port=4
  dphi_load [rad/s] x4 : Inport  Port=5
  dphi_motor [rad/s] x4 : Inport  Port=6
  % of critical damping : Subsystem
  Constant : Constant  Value=ctrl.kp_sea
  Product2 : Product  RndMeth=Zero
  Spring Stiffness : Gain  Gain=ctrl.k_sea
  Spring Stiffness 1 : Gain  Gain=ctrl.k_sea
  Sum1 : Sum  Inputs=-+|
  Sum2 : Sum  Inputs=|+-
  Sum3 : Sum  Inputs=++|
  Sum5 : Sum  Inputs=|+-
  Sum6 : Sum  Inputs=-+|
  Sum7 : Sum  Inputs=+|+
  kp_sea : Gain  Gain=ctrl.kp_sea
  tau_cmd sagittal [Nm] x4 : Outport
  tau_measured [Nm] x4 : Outport  Port=2
  wires:
  % of critical damping/1(d gain) -> Product2/1
  Sum3/1 -> tau_cmd sagittal [Nm] x4/1
  Sum7/1 -> Sum3/2
  Spring Stiffness/1 -> tau_measured [Nm] x4/1, Sum5/2
  Sum1/1 -> Spring Stiffness/1
  phi_load [rad] x4/1 -> Sum1/1
  phi_motor [rad] x4/1 -> Sum1/2
  tau_des sagittal [Nm] x4/1 -> Sum3/1, Sum5/1
  dtau_des sagittal [Nm] x4/1 -> Sum2/1
  Sum6/1 -> Spring Stiffness 1/1
  Spring Stiffness 1/1 -> Sum2/2
  dphi_load [rad/s] x4/1 -> Sum6/1
  dphi_motor [rad/s] x4/1 -> Sum6/2
  Sum5/1 -> kp_sea/1
  Sum2/1 -> Product2/2
  Product2/1 -> Sum7/2
  kp_sea/1 -> Sum7/1
  Constant/1 -> % of critical damping/1(p gain)
